simulink model "msk_simu"  (R2019b)
settings: Solver=VariableStepAuto  StartTime=0.0  StopTime=10.0  RelTol=1e-3
libraries: commdigbbndpm3 x2, commchan3 x1, commsink2 x1, commutil2 x1, commrandsrc3 x1
settings Model: Creator=yango  LastModifiedBy=yango

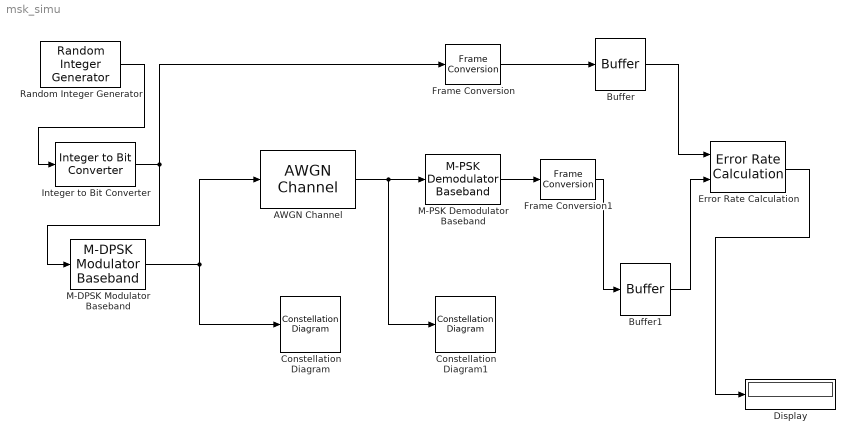
== system msk_simu ==
  AWGN Channel : commchan3/AWGN Channel  InputProcessing=Columns as channels (frame based)  seed=67  noiseMode="Signal to noise ratio  (Eb/No)"  EbNodB=15  EsNodB=10  SNRdB=10  bitsPerSym=3  Ps=1  Tsym=1/1000  variance=1
      settings: SourceProductName=Communications Toolbox
  Buffer : Buffer  OutputFrames=off
  Buffer1 : Buffer  OutputFrames=off
  Constellation Diagram : ConstellationDiagram
  Constellation Diagram1 : ConstellationDiagram
  Display : Display
  Error Rate Calculation : commsink2/Error Rate Calculation  N=0  st_delay=0  cp_mode=Entire frame  subframe=[]  PMode=Port  WsName=ErrorVec  RsMode2=off  stop=off  numErr=100  maxBits=1e6
      settings: SourceProductName=Communications Toolbox
  Frame Conversion : FrameConversion
  Frame Conversion1 : FrameConversion
  Integer to Bit Converter : commutil2/Integer to Bit Converter  nbits=3  signedInputValues=Unsigned  bitOrder=MSB first  outDtype=Inherit via internal rule
      settings: SourceProductName=Communications Toolbox
  M-DPSK Modulator Baseband : commdigbbndpm3/M-DPSK Modulator Baseband  M=8  InType=Bit  Enc=Gray  Ph=pi/8  outDtype=double
      settings: SourceProductName=Communications Toolbox  SourceProductBaseCode=CM
  M-PSK Demodulator Baseband : commdigbbndpm3/M-PSK Demodulator Baseband  M=8  OutType=Bit  DecType=Hard decision  VarSource=Dialog  Variance=1  Dec=Gray  Mapping=[0:7]  Ph=pi/8  outDtype1=Inherit via internal rule  outDtype2=Inherit via internal rule  derotateFactorWordLen=16  derotateFactorDataTypeStr=Inherit: Same word length as input  derotateFactorLastDataTypeStr=Inherit: Same word length as input
      settings: SourceProductName=Communications Toolbox
  Random Integer Generator : commrandsrc3/Random Integer Generator  SetSize=8  SeedSource=Auto  Seed=0  SampleTime=1/1000  SamplesPerFrame=1  OutputDataType=uint8  SimulateUsing=Interpreted execution
      settings: SourceProductName=Communications Toolbox
  wires:
  Random Integer Generator/1 -> Integer to Bit Converter/1
  Integer to Bit Converter/1 -> M-DPSK Modulator Baseband/1, Frame Conversion/1
  M-DPSK Modulator Baseband/1 -> Constellation Diagram/1, AWGN Channel/1
  AWGN Channel/1 -> Constellation Diagram1/1, M-PSK Demodulator Baseband/1
  Frame Conversion/1 -> Buffer/1
  M-PSK Demodulator Baseband/1 -> Frame Conversion1/1
  Buffer/1 -> Error Rate Calculation/1
  Error Rate Calculation/1 -> Display/1
  Buffer1/1 -> Error Rate Calculation/2
  Frame Conversion1/1 -> Buffer1/1
